simulink model "iter_imas_contr_4"  (Simulink 8.5)
settings: Solver=ode1  StartTime=EqTime  StopTime=1e8  FixedStep=SimStep  MaxStep=5.e-3  MinStep=2e-4  RelTol=1.e-3
undefined symbols (not defined in the file): Elong, g1, g1_term, g2, g2_term, g3, g3_term, g4, g4_term, g5, g5_term, g6, g6_term, Imax, key_imas, n_gaps, n_mc, ncam, npf, ntur, RupRd, scr_data, SimStep, Vcspf_up, vec_imas, volt
libraries: simulink x56
(part 2 of 3)

== system iter_imas_contr_4/kavin_contr/Control inputs 1/err(Ic) scr_data.dat/Icoil2 ref ==
  Time : Inport
  eob : Inport  Port=2
  Divide1 : Product  Inputs=**
  I1 : simulink/Lookup Tables/Lookup Table Dynamic  LookUpMeth=Interpolation-Use End Values  OutDataTypeStr=fixdt('double')  OutputDataTypeScalingMode=Specify via dialog  OutDataType=fixdt('double')  OutScaling=2^-10  DoSatur=off
  Memory2 : Memory
  c_eob : Switch  Threshold=1
  scr1 Read : DataStoreRead  DataStoreName=scr_data  DataStoreElements=scr_data(1,:)
  scr2 Read : DataStoreRead  DataStoreName=scr_data  DataStoreElements=scr_data(4,:)
  " " : Outport
  wires:
  c_eob/1 -> Memory2/1, Divide1/1
  Divide1/1 -> " "/1
  Time/1 -> I1/1
  eob/1 -> c_eob/2, Divide1/2
  Memory2/1 -> c_eob/3
  scr2 Read/1 -> I1/3
  I1/1 -> c_eob/1
  scr1 Read/1 -> I1/2

== system iter_imas_contr_4/kavin_contr/Control inputs 1/err(Ic) scr_data.dat/Icoil3 ref ==
  Time : Inport
  eob : Inport  Port=2
  Divide1 : Product  Inputs=**
  I1 : simulink/Lookup Tables/Lookup Table Dynamic  LookUpMeth=Interpolation-Use End Values  OutDataTypeStr=fixdt('double')  OutputDataTypeScalingMode=Specify via dialog  OutDataType=fixdt('double')  OutScaling=2^-10  DoSatur=off
  Memory2 : Memory
  c_eob : Switch  Threshold=1
  scr1 Read : DataStoreRead  DataStoreName=scr_data  DataStoreElements=scr_data(1,:)
  scr5 Read : DataStoreRead  DataStoreName=scr_data  DataStoreElements=scr_data(5,:)
  " " : Outport
  wires:
  c_eob/1 -> Memory2/1, Divide1/1
  Divide1/1 -> " "/1
  Time/1 -> I1/1
  eob/1 -> c_eob/2, Divide1/2
  Memory2/1 -> c_eob/3
  scr5 Read/1 -> I1/3
  I1/1 -> c_eob/1
  scr1 Read/1 -> I1/2

== system iter_imas_contr_4/kavin_contr/Control inputs 1/err(Ic) scr_data.dat/Icoil4 ref ==
  Time : Inport
  eob : Inport  Port=2
  Divide1 : Product  Inputs=**
  I1 : simulink/Lookup Tables/Lookup Table Dynamic  LookUpMeth=Interpolation-Use End Values  OutDataTypeStr=fixdt('double')  OutputDataTypeScalingMode=Specify via dialog  OutDataType=fixdt('double')  OutScaling=2^-10  DoSatur=off
  Memory2 : Memory
  c_eob : Switch  Threshold=1
  scr1 Read : DataStoreRead  DataStoreName=scr_data  DataStoreElements=scr_data(1,:)
  scr6 Read : DataStoreRead  DataStoreName=scr_data  DataStoreElements=scr_data(6,:)
  " " : Outport
  wires:
  c_eob/1 -> Memory2/1, Divide1/1
  Divide1/1 -> " "/1
  Time/1 -> I1/1
  eob/1 -> c_eob/2, Divide1/2
  Memory2/1 -> c_eob/3
  scr6 Read/1 -> I1/3
  I1/1 -> c_eob/1
  scr1 Read/1 -> I1/2

== system iter_imas_contr_4/kavin_contr/Control inputs 1/err(Ic) scr_data.dat/Icoil5 ref ==
  Time : Inport
  eob : Inport  Port=2
  Divide1 : Product  Inputs=**
  I1 : simulink/Lookup Tables/Lookup Table Dynamic  LookUpMeth=Interpolation-Use End Values  OutDataTypeStr=fixdt('double')  OutputDataTypeScalingMode=Specify via dialog  OutDataType=fixdt('double')  OutScaling=2^-10  DoSatur=off
  Memory2 : Memory
  c_eob : Switch  Threshold=1
  scr1 Read : DataStoreRead  DataStoreName=scr_data  DataStoreElements=scr_data(1,:)
  scr7 Read : DataStoreRead  DataStoreName=scr_data  DataStoreElements=scr_data(7,:)
  " " : Outport
  wires:
  c_eob/1 -> Memory2/1, Divide1/1
  Divide1/1 -> " "/1
  Time/1 -> I1/1
  eob/1 -> c_eob/2, Divide1/2
  Memory2/1 -> c_eob/3
  scr7 Read/1 -> I1/3
  I1/1 -> c_eob/1
  scr1 Read/1 -> I1/2

== system iter_imas_contr_4/kavin_contr/Control inputs 1/err(Ic) scr_data.dat/Icoil6 ref ==
  Time : Inport
  eob : Inport  Port=2
  Divide1 : Product  Inputs=**
  I1 : simulink/Lookup Tables/Lookup Table Dynamic  LookUpMeth=Interpolation-Use End Values  OutDataTypeStr=fixdt('double')  OutputDataTypeScalingMode=Specify via dialog  OutDataType=fixdt('double')  OutScaling=2^-10  DoSatur=off
  Memory2 : Memory
  c_eob : Switch  Threshold=1
  scr8 Read : DataStoreRead  DataStoreName=scr_data  DataStoreElements=scr_data(8,:)
  sct1 Read : DataStoreRead  DataStoreName=scr_data  DataStoreElements=scr_data(1,:)
  "  " : Outport
  wires:
  c_eob/1 -> Divide1/1, Memory2/1
  Divide1/1 -> "  "/1
  Time/1 -> I1/1
  eob/1 -> Divide1/2, c_eob/2
  Memory2/1 -> c_eob/3
  scr8 Read/1 -> I1/3
  I1/1 -> c_eob/1
  sct1 Read/1 -> I1/2

== system iter_imas_contr_4/kavin_contr/Control inputs 1/err(Ic) scr_data.dat/Icoil7 ref ==
  Time : Inport
  eob : Inport  Port=2
  Divide1 : Product  Inputs=**
  I1 : simulink/Lookup Tables/Lookup Table Dynamic  LookUpMeth=Interpolation-Use End Values  OutDataTypeStr=fixdt('double')  OutputDataTypeScalingMode=Specify via dialog  OutDataType=fixdt('double')  OutScaling=2^-10  DoSatur=off
  Memory2 : Memory
  c_eob : Switch  Threshold=1
  scr1 Read : DataStoreRead  DataStoreName=scr_data  DataStoreElements=scr_data(1,:)
  scr9 Read : DataStoreRead  DataStoreName=scr_data  DataStoreElements=scr_data(9,:)
  " " : Outport
  wires:
  c_eob/1 -> Divide1/1, Memory2/1
  Divide1/1 -> " "/1
  Time/1 -> I1/1
  eob/1 -> c_eob/2, Divide1/2
  Memory2/1 -> c_eob/3
  scr9 Read/1 -> I1/3
  I1/1 -> c_eob/1
  scr1 Read/1 -> I1/2

== system iter_imas_contr_4/kavin_contr/Control inputs 1/err(Ic) scr_data.dat/Icoil8 ref ==
  Time : Inport
  eob : Inport  Port=2
  Divide1 : Product  Inputs=**
  I1 : simulink/Lookup Tables/Lookup Table Dynamic  LookUpMeth=Interpolation-Use End Values  OutDataTypeStr=fixdt('double')  OutputDataTypeScalingMode=Specify via dialog  OutDataType=fixdt('double')  OutScaling=2^-10  DoSatur=off
  Memory2 : Memory
  c_eob : Switch  Threshold=1
  scr1 Read : DataStoreRead  DataStoreName=scr_data  DataStoreElements=scr_data(1,:)
  scr10 Read : DataStoreRead  DataStoreName=scr_data  DataStoreElements=scr_data(10,:)
  "  " : Outport
  wires:
  c_eob/1 -> Divide1/1, Memory2/1
  Divide1/1 -> "  "/1
  Time/1 -> I1/1
  eob/1 -> c_eob/2, Divide1/2
  Memory2/1 -> c_eob/3
  scr10 Read/1 -> I1/3
  I1/1 -> c_eob/1
  scr1 Read/1 -> I1/2

== system iter_imas_contr_4/kavin_contr/Control inputs 1/err(Ic) scr_data.dat/Icoil9 ref ==
  Time : Inport
  eob : Inport  Port=2
  Divide1 : Product  Inputs=**
  I1 : simulink/Lookup Tables/Lookup Table Dynamic  LookUpMeth=Interpolation-Use End Values  OutDataTypeStr=fixdt('double')  OutputDataTypeScalingMode=Specify via dialog  OutDataType=fixdt('double')  OutScaling=2^-10  DoSatur=off
  Memory2 : Memory
  c_eob : Switch  Threshold=1
  scr1 Read : DataStoreRead  DataStoreName=scr_data  DataStoreElements=scr_data(1,:)
  scr11 Read : DataStoreRead  DataStoreName=scr_data  DataStoreElements=scr_data(11,:)
  " " : Outport
  wires:
  c_eob/1 -> Divide1/1, Memory2/1
  Divide1/1 -> " "/1
  Time/1 -> I1/1
  eob/1 -> Divide1/2, c_eob/2
  Memory2/1 -> c_eob/3
  scr11 Read/1 -> I1/3
  I1/1 -> c_eob/1
  scr1 Read/1 -> I1/2

== system iter_imas_contr_4/kavin_contr/Control inputs 1/g1-g6.dat,g1_term-g6_term.dat/g1 ==
  Time : Inport
  eob : Inport  Port=2
  Memory1 : Memory
  Memory2 : Memory
  c_eob : Switch  Threshold=1
  "c_eob  " : Switch  Threshold=1
  c_eob  1 : Switch  Threshold=1
  g1 Read : DataStoreRead  DataStoreName=g1  DataStoreElements=g1(1,:)
  g1 Read1 : DataStoreRead  DataStoreName=g1  DataStoreElements=g1(2,:)
  g1_term,ref : Subsystem
  g1ref1 : simulink/Lookup Tables/Lookup Table Dynamic  LookUpMeth=Interpolation-Use End Values  OutDataTypeStr=fixdt('double')  OutputDataTypeScalingMode=Specify via dialog  OutDataType=fixdt('double')  OutScaling=2^-10  DoSatur=off
  Out1 : Outport
  wires:
  eob/1 -> "c_eob  "/2, c_eob/2, c_eob  1/2
  Memory1/1 -> "c_eob  "/3
  "c_eob  "/1 -> Memory1/1, g1_term,ref/3(Time_eob)
  g1_term,ref/1(Out1) -> c_eob/3
  c_eob/1 -> Out1/1
  Time/1 -> g1ref1/1, g1_term,ref/2(Time), "c_eob  "/1
  g1ref1/1 -> c_eob  1/1
  Memory2/1 -> c_eob  1/3
  c_eob  1/1 -> g1_term,ref/1(g1ref_eob), Memory2/1, c_eob/1
  g1 Read/1 -> g1ref1/2
  g1 Read1/1 -> g1ref1/3

== system iter_imas_contr_4/kavin_contr/Control inputs 1/g1-g6.dat,g1_term-g6_term.dat/g2 ==
  Time : Inport
  eob : Inport  Port=2
  Memory1 : Memory
  Memory2 : Memory
  c_eob : Switch  Threshold=1
  "c_eob  " : Switch  Threshold=1
  c_eob  1 : Switch  Threshold=1
  g2 Read : DataStoreRead  DataStoreName=g2  DataStoreElements=g2(1,:)
  g2 Read1 : DataStoreRead  DataStoreName=g2  DataStoreElements=g2(2,:)
  g2_term,ref : Subsystem
  g2ref : simulink/Lookup Tables/Lookup Table Dynamic  LookUpMeth=Interpolation-Use End Values  OutDataTypeStr=fixdt('double')  OutputDataTypeScalingMode=Specify via dialog  OutDataType=fixdt('double')  OutScaling=2^-10  DoSatur=off
  Out1 : Outport
  wires:
  eob/1 -> "c_eob  "/2, c_eob  1/2, c_eob/2
  Memory1/1 -> "c_eob  "/3
  "c_eob  "/1 -> g2_term,ref/3(Time_eob), Memory1/1
  g2_term,ref/1(Out1) -> c_eob/3
  c_eob/1 -> Out1/1
  g2 Read1/1 -> g2ref/3
  g2 Read/1 -> g2ref/2
  Time/1 -> g2ref/1, "c_eob  "/1, g2_term,ref/2(Time)
  g2ref/1 -> c_eob  1/1
  Memory2/1 -> c_eob  1/3
  c_eob  1/1 -> g2_term,ref/1(g2ref_eob), Memory2/1, c_eob/1

== system iter_imas_contr_4/kavin_contr/Control inputs 1/g1-g6.dat,g1_term-g6_term.dat/g3 ==
  Time : Inport
  eob : Inport  Port=2
  Memory1 : Memory
  Memory2 : Memory
  c_eob : Switch  Threshold=1
  "c_eob  " : Switch  Threshold=1
  c_eob  1 : Switch  Threshold=1
  g3 Read : DataStoreRead  DataStoreName=g3  DataStoreElements=g3(1,:)
  g3 Read1 : DataStoreRead  DataStoreName=g3  DataStoreElements=g3(2,:)
  g3_term,ref : Subsystem
  g3ref : simulink/Lookup Tables/Lookup Table Dynamic  LookUpMeth=Interpolation-Use End Values  OutDataTypeStr=fixdt('double')  OutputDataTypeScalingMode=Specify via dialog  OutDataType=fixdt('double')  OutScaling=2^-10  DoSatur=off
  Out1 : Outport
  wires:
  eob/1 -> "c_eob  "/2, c_eob/2, c_eob  1/2
  Memory1/1 -> "c_eob  "/3
  "c_eob  "/1 -> g3_term,ref/3(Time_eob), Memory1/1
  g3_term,ref/1(Out1) -> c_eob/3
  c_eob/1 -> Out1/1
  Time/1 -> g3ref/1, "c_eob  "/1, g3_term,ref/2(Time)
  g3ref/1 -> c_eob  1/1
  c_eob  1/1 -> g3_term,ref/1(g3ref_eob), Memory2/1, c_eob/1
  Memory2/1 -> c_eob  1/3
  g3 Read/1 -> g3ref/2
  g3 Read1/1 -> g3ref/3

== system iter_imas_contr_4/kavin_contr/Control inputs 1/g1-g6.dat,g1_term-g6_term.dat/g4 ==
  Time : Inport
  eob : Inport  Port=2
  Memory1 : Memory
  Memory2 : Memory
  c_eob : Switch  Threshold=1
  "c_eob  " : Switch  Threshold=1
  c_eob  1 : Switch  Threshold=1
  g4 Read : DataStoreRead  DataStoreName=g4  DataStoreElements=g4(1,:)
  g4 Read1 : DataStoreRead  DataStoreName=g4  DataStoreElements=g4(2,:)
  g4_term,ref : Subsystem
  g4ref : simulink/Lookup Tables/Lookup Table Dynamic  LookUpMeth=Interpolation-Use End Values  OutDataTypeStr=fixdt('double')  OutputDataTypeScalingMode=Specify via dialog  OutDataType=fixdt('double')  OutScaling=2^-10  DoSatur=off
  Out1 : Outport
  wires:
  eob/1 -> "c_eob  "/2, c_eob/2, c_eob  1/2
  Memory1/1 -> "c_eob  "/3
  "c_eob  "/1 -> Memory1/1, g4_term,ref/3(Time_eob)
  g4_term,ref/1(Out1) -> c_eob/3
  c_eob/1 -> Out1/1
  Time/1 -> g4ref/1, "c_eob  "/1, g4_term,ref/2(Time)
  g4ref/1 -> c_eob  1/1
  Memory2/1 -> c_eob  1/3
  c_eob  1/1 -> g4_term,ref/1(g4ref_eob), Memory2/1, c_eob/1
  g4 Read/1 -> g4ref/2
  g4 Read1/1 -> g4ref/3

== system iter_imas_contr_4/kavin_contr/Control inputs 1/g1-g6.dat,g1_term-g6_term.dat/g5 ==
  Time : Inport
  eob : Inport  Port=2
  Memory1 : Memory
  Memory2 : Memory
  c_eob : Switch  Threshold=1
  "c_eob  " : Switch  Threshold=1
  c_eob  1 : Switch  Threshold=1
  g5 Read : DataStoreRead  DataStoreName=g5  DataStoreElements=g5(1,:)
  g5 Read1 : DataStoreRead  DataStoreName=g5  DataStoreElements=g5(2,:)
  g5_term,ref : Subsystem
  g5ref : simulink/Lookup Tables/Lookup Table Dynamic  LookUpMeth=Interpolation-Use End Values  OutDataTypeStr=fixdt('double')  OutputDataTypeScalingMode=Specify via dialog  OutDataType=fixdt('double')  OutScaling=2^-10  DoSatur=off
  Out1 : Outport
  wires:
  eob/1 -> c_eob  1/2, "c_eob  "/2, c_eob/2
  Memory1/1 -> "c_eob  "/3
  "c_eob  "/1 -> Memory1/1, g5_term,ref/3(Time_eob)
  g5_term,ref/1(Out1) -> c_eob/3
  c_eob/1 -> Out1/1
  Time/1 -> g5ref/1, "c_eob  "/1, g5_term,ref/2(Time)
  g5ref/1 -> c_eob  1/1
  c_eob  1/1 -> Memory2/1, g5_term,ref/1(g5ref_eob), c_eob/1
  Memory2/1 -> c_eob  1/3
  g5 Read/1 -> g5ref/2
  g5 Read1/1 -> g5ref/3

== system iter_imas_contr_4/kavin_contr/Control inputs 1/g1-g6.dat,g1_term-g6_term.dat/g6 ==
  Time : Inport
  eob : Inport  Port=2
  Memory1 : Memory
  Memory2 : Memory
  c_eob : Switch  Threshold=1
  "c_eob  " : Switch  Threshold=1
  c_eob  1 : Switch  Threshold=1
  g6 Read : DataStoreRead  DataStoreName=g6  DataStoreElements=g6(1,:)
  g6 Read1 : DataStoreRead  DataStoreName=g6  DataStoreElements=g6(2,:)
  g6_term,ref : Subsystem
  g6ref : simulink/Lookup Tables/Lookup Table Dynamic  LookUpMeth=Interpolation-Use End Values  OutDataTypeStr=fixdt('double')  OutputDataTypeScalingMode=Specify via dialog  OutDataType=fixdt('double')  OutScaling=2^-10  DoSatur=off
  Out1 : Outport
  wires:
  eob/1 -> "c_eob  "/2, c_eob  1/2, c_eob/2
  Memory1/1 -> "c_eob  "/3
  "c_eob  "/1 -> Memory1/1, g6_term,ref/3(Time_eob)
  g6_term,ref/1(Out1) -> c_eob/3
  c_eob/1 -> Out1/1
  Time/1 -> g6ref/1, "c_eob  "/1, g6_term,ref/2(Time)
  g6ref/1 -> c_eob  1/1
  c_eob  1/1 -> g6_term,ref/1(g6ref_eob), Memory2/1, c_eob/1
  Memory2/1 -> c_eob  1/3
  g6 Read/1 -> g6ref/2
  g6 Read1/1 -> g6ref/3

== system iter_imas_contr_4/kavin_contr/Control inputs 1/trd/If Action Subsystem2 ==
  "time " : Inport
  Action Port : ActionPort  ActionType=then
  Data Store Write2 : DataStoreWrite  DataStoreName=trd
  wires:
  "time "/1 -> Data Store Write2/1

== system iter_imas_contr_4/kavin_contr/Control inputs 1/trd/Trigger ==
  Input : Inport
  Logical Operator : Logic  Operator=OR  AllPortsSameDT=off  OutDataTypeStr=float('double')
  Memory : Memory
  State : Outport
  wires:
  Memory/1 -> Logical Operator/2
  Input/1 -> Logical Operator/1
  Logical Operator/1 -> State/1, Memory/1

== system iter_imas_contr_4/kavin_contr/Control inputs 1/tterm/If Action Subsystem2 ==
  "time " : Inport
  Action Port : ActionPort  ActionType=then
  Data Store Write2 : DataStoreWrite  DataStoreName=tterm
  wires:
  "time "/1 -> Data Store Write2/1

== system iter_imas_contr_4/kavin_contr/Control inputs 1/tterm/Ip<cIp_end ==
  Ip : Inport
  Abs : Abs
  Data Store Read : DataStoreRead  DataStoreName=RupRd  DataStoreElements=RupRd(3)
  Relational Operator : RelationalOperator  Operator=<  OutDataTypeStr=boolean
  Out1 : Outport
  wires:
  Data Store Read/1 -> Abs/1
  Ip/1 -> Relational Operator/1
  Abs/1 -> Relational Operator/2
  Relational Operator/1 -> Out1/1

== system iter_imas_contr_4/kavin_contr/Control inputs 1/tterm/Trigger ==
  Input : Inport
  Logical Operator : Logic  Operator=OR  AllPortsSameDT=off  OutDataTypeStr=float('double')
  Memory : Memory
  State : Outport
  wires:
  Memory/1 -> Logical Operator/2
  Input/1 -> Logical Operator/1
  Logical Operator/1 -> State/1, Memory/1

== system iter_imas_contr_4/kavin_contr/Control1/VS control/Ip>cIp_end ==
  time : Inport
  Data Store Read2 : DataStoreRead  DataStoreName=tterm
  Relational Operator2 : RelationalOperator  Operator=<  OutDataTypeStr=float('double')
  1 or 0 : Outport
  wires:
  time/1 -> Relational Operator2/1
  Relational Operator2/1 -> 1 or 0/1
  Data Store Read2/1 -> Relational Operator2/2

== system iter_imas_contr_4/kavin_contr/Control1/VS control/dzdt noise1 ==
  VS3 inputs : Inport
  Time : Inport  Port=2
  Demux : Demux  Outputs=[1 1]
  Mux : Mux  Inputs=2
  Subsystem : Subsystem
  Sum2 : Sum
  Uniform Random Number : UniformRandomNumber  SampleTime=SimStep
  Out1 : Outport
  wires:
  VS3 inputs/1 -> Demux/1
  Demux/1 -> Sum2/2
  Sum2/1 -> Mux/1
  Demux/2 -> Mux/2
  Mux/1 -> Out1/1
  Uniform Random Number/1 -> Subsystem/1(Noise)
  Time/1 -> Subsystem/2(Time)
  Subsystem/1(Out1) -> Sum2/1

== system iter_imas_contr_4/kavin_contr/Control1/VS control/eob < 1 ==
  note: Ip<Ip_rd
  note: Ip>Ip_rd
  err VS : Inport
  Ip : Inport  Port=2
  "eob " : Inport  Port=3
  "time " : Inport  Port=4
  Compare To Constant1 : simulink/Logic and Bit Operations/Compare To Constant  relop=<  const=1  OutDataTypeStr=boolean  ZeroCross=off
  Divide1 : Product  Inputs=**
  Divide4 : Product  Inputs=**
  Ip < Ip_rd : Subsystem
  Ip > Ip_rd : Subsystem
  "Ip_rd " : Switch  Threshold=1
  Ip_rd tr : Subsystem
  VS. contr hl : Subsystem
  Out1 : Outport
  wires:
  Ip < Ip_rd/1(Out1) -> "Ip_rd "/1
  Ip > Ip_rd/1(Out1) -> "Ip_rd "/3
  Ip/1 -> Ip < Ip_rd/1(Ip), Ip > Ip_rd/1(Ip)
  Divide1/1 -> Out1/1
  VS. contr hl/1(Out1) -> Divide1/1
  "Ip_rd "/1 -> Divide1/2
  err VS/1 -> Divide4/1
  Divide4/1 -> VS. contr hl/1(In1)
  "eob "/1 -> Compare To Constant1/1, Ip_rd tr/2("eob ")
  Compare To Constant1/1 -> Divide4/2
  "time "/1 -> Ip_rd tr/1(Time)
  Ip_rd tr/1(0 or 1) -> "Ip_rd "/2

== system iter_imas_contr_4/kavin_contr/Control1/VS control/eob >= 1 ==
  Ipl : Inport
  time : Inport  Port=2
  err VS : Inport  Port=3
  Divide8 : Product  Inputs=**
  VS. contr1 : Subsystem
  dim or lim : Subsystem
  Out1 : Outport
  wires:
  err VS/1 -> VS. contr1/1(In1)
  Ipl/1 -> dim or lim/1(Ipl)
  time/1 -> dim or lim/2(Time)
  dim or lim/1(VS gain) -> Divide8/1
  VS. contr1/1(Out1) -> Divide8/2
  Divide8/1 -> Out1/1

== system iter_imas_contr_4/kavin_contr/Control1/VS control/t_tran2D ==
  Noise,VS3 : Inport
  Time : Inport  Port=2
  Data Store Read : DataStoreRead  DataStoreName=t_tran2D  DataStoreElements=t_tran2D
  Divide12 : Product  Inputs=**
  Relational Operator1 : RelationalOperator  Operator=>  OutDataTypeStr=float('double')
  Out1 : Outport
  wires:
  Noise,VS3/1 -> Divide12/1
  Time/1 -> Relational Operator1/1
  Data Store Read/1 -> Relational Operator1/2
  Relational Operator1/1 -> Divide12/2
  Divide12/1 -> Out1/1

== system iter_imas_contr_4/kavin_contr/Control1/controllers/ tt_kavin2.dat(1) ==
  Time : Inport
  1 : Constant
  Data Store Read : DataStoreRead  DataStoreName=ref_ramp  DataStoreElements=ref_ramp
  Data Store Read1 : DataStoreRead  DataStoreName=tdiv  DataStoreElements=tdiv
  Divide1 : Product  Inputs=/*
  Memory3 : Memory
  Relational Operator1 : RelationalOperator  OutDataTypeStr=float('double')
  Saturation1 : Saturate  UpperLimit=1  LowerLimit=0
  Subtract1 : Sum
  Subtract2 : Sum  Inputs=+-
  Subtract3 : Sum  Inputs=+-
  "switch1 " : Switch  Threshold=1
  1-0 : Outport
  0-1 : Outport  Port=2
  wires:
  "switch1 "/1 -> Memory3/1, Subtract2/1
  Memory3/1 -> "switch1 "/1
  Subtract2/1 -> Divide1/2
  Divide1/1 -> Subtract1/1
  Subtract1/1 -> Saturation1/1
  Saturation1/1 -> Subtract3/2, 1-0/1
  1/1 -> Subtract1/2, Subtract3/1
  Time/1 -> "switch1 "/3, Subtract2/2, Relational Operator1/1
  Data Store Read/1 -> Divide1/1
  Relational Operator1/1 -> "switch1 "/2
  Subtract3/1 -> 0-1/1
  Data Store Read1/1 -> Relational Operator1/2

== system iter_imas_contr_4/kavin_contr/Control1/controllers/Div rd contr ==
  gain : Inport
  time : Inport  Port=2
  err : Inport  Port=3
  Div_rd contr : Subsystem
  Divide3 : Product  Inputs=**
  Divide4 : Product  Inputs=**
  div_rd tr : Subsystem
  Div rd volt : Outport
  wires:
  gain/1 -> Divide3/1
  err/1 -> Divide4/2
  time/1 -> div_rd tr/1("time ")
  Divide3/1 -> Div rd volt/1
  Div_rd contr/1(Out1) -> Divide3/2
  Divide4/1 -> Div_rd contr/1(In1)
  div_rd tr/1(0 or 1) -> Divide4/1

== system iter_imas_contr_4/kavin_contr/Control1/controllers/Div. contr ==
  time : Inport
  err : Inport  Port=2
  gain : Inport  Port=3
  Div. contr. : Subsystem
  Divide : Product  Inputs=**
  Divide2 : Product  Inputs=**
  Udiv : Subsystem
  div tr : Subsystem
  "Div volt " : Outport
  wires:
  Udiv/1("Udiv ") -> "Div volt "/1
  Divide/1 -> Udiv/1(Udiv)
  div tr/1("0 or 1 ") -> Divide2/1
  Div. contr./1(Out1) -> Divide/1
  Divide2/1 -> Div. contr./1(In1)
  time/1 -> div tr/1(Time), Udiv/2("time ")
  err/1 -> Divide2/2
  gain/1 -> Divide/2

== system iter_imas_contr_4/kavin_contr/Control1/controllers/Ip>cIp_end1 ==
  Time : Inport
  1 : Constant
  "1 " : Switch  Threshold=1
  Data Store Read : DataStoreRead  DataStoreName=ref_ramp  DataStoreElements=ref_ramp
  Data Store Read2 : DataStoreRead  DataStoreName=tterm
  Divide4 : Product  Inputs=/*
  Memory1 : Memory
  Relational Operator2 : RelationalOperator  OutDataTypeStr=float('double')
  Saturation : Saturate  UpperLimit=1  LowerLimit=0
  Subtract1 : Sum  Inputs=-+
  Subtract2 : Sum  Inputs=+-
  Subtract3 : Sum
  1-0 : Outport
  0-1 : Outport  Port=2
  wires:
  Time/1 -> Subtract2/2, "1 "/3, Relational Operator2/1
  "1 "/1 -> Memory1/1, Subtract2/1
  Memory1/1 -> "1 "/1
  Subtract2/1 -> Divide4/2
  Divide4/1 -> Subtract3/1
  1/1 -> Subtract3/2, Subtract1/2
  Subtract3/1 -> Saturation/1
  Subtract1/1 -> 0-1/1
  Saturation/1 -> 1-0/1, Subtract1/1
  Data Store Read/1 -> Divide4/1
  Relational Operator2/1 -> "1 "/2
  Data Store Read2/1 -> Relational Operator2/2

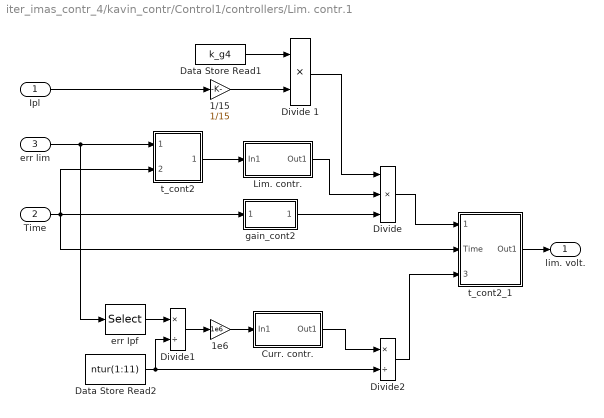
== system iter_imas_contr_4/kavin_contr/Control1/controllers/Lim. contr.1 ==
  Ipl : Inport
  Time : Inport  Port=2
  err lim : Inport  Port=3
  1/15 : Gain  Gain=1/15
  1e6 : Gain  Gain=1e6
  Curr. contr. : Subsystem
  Data Store Read1 : DataStoreRead  DataStoreName=k_g4  DataStoreElements=k_g4
  Data Store Read2 : DataStoreRead  DataStoreName=ntur  DataStoreElements=ntur(1:11)
  "Divide " : Product  Inputs=***
  Divide 1 : Product  Inputs=**
  Divide1 : Product  Inputs=*/
  Divide2 : Product  Inputs=*/
  Lim. contr. : Subsystem
  err Ipf : Selector  InputPortWidth=20  Indices=[9:19]
  gain_cont2 : Subsystem
  t_cont2 : Subsystem
  t_cont2_1 : Subsystem
  lim. volt. : Outport
  wires:
  err lim/1 -> err Ipf/1, t_cont2/1(errlim)
  Time/1 -> t_cont2_1/2(Time), gain_cont2/1(Time), t_cont2/2(Time)
  Divide1/1 -> 1e6/1
  Curr. contr./1(Out1) -> Divide2/1
  t_cont2/1(Out1) -> Lim. contr./1(In1)
  err Ipf/1 -> Divide1/1
  Data Store Read2/1 -> Divide1/2, Divide2/2
  "Divide "/1 -> t_cont2_1/1(lim. contr.)
  Divide2/1 -> t_cont2_1/3(Curr. cont.)
  t_cont2_1/1(Out1) -> lim. volt./1
  1e6/1 -> Curr. contr./1(In1)
  gain_cont2/1(Out1) -> "Divide "/3
  Lim. contr./1(Out1) -> "Divide "/2
  Ipl/1 -> 1/15/1
  Divide 1/1 -> "Divide "/1
  Data Store Read1/1 -> Divide 1/1
  1/15/1 -> Divide 1/2

== system iter_imas_contr_4/kavin_contr/Control1/controllers/curr term contr ==
  Time : Inport
  Icoil : Inport  Port=2
  " G_curr_term 1" : Gain  Gain=[zeros(8,11); eye(11); zeros(1,11)]  Multiplication=Matrix(K*u)
  Curr. term. contr : Subsystem
  Divide12 : Product  Inputs=**
  term tr : Subsystem
  term volt : Outport
  wires:
  Curr. term. contr/1(Out1) -> term volt/1
  Divide12/1 -> Curr. term. contr/1(In1)
  " G_curr_term 1"/1 -> Divide12/1
  Icoil/1 -> " G_curr_term 1"/1
  Time/1 -> term tr/1(Time)
  term tr/1(Out1) -> Divide12/2

== system iter_imas_contr_4/kavin_contr/Control1/controllers/div_divrd ==
  Time : Inport
  1 : Constant
  Data Store Read1 : DataStoreRead  DataStoreName=ref_ramp  DataStoreElements=ref_ramp
  Data Store Read2 : DataStoreRead  DataStoreName=trd
  Divide4 : Product  Inputs=/*
  Memory1 : Memory
  Relational Operator2 : RelationalOperator  OutDataTypeStr=float('double')
  Saturation : Saturate  UpperLimit=1  LowerLimit=0
  Subtract1 : Sum  Inputs=+-
  Subtract2 : Sum  Inputs=+-
  Subtract3 : Sum
  switch1 : Switch  Threshold=1
  1-0 : Outport
  0-1 : Outport  Port=2
  wires:
  switch1/1 -> Subtract2/1, Memory1/1
  Memory1/1 -> switch1/1
  Subtract2/1 -> Divide4/2
  Divide4/1 -> Subtract3/1
  Subtract3/1 -> Saturation/1
  Saturation/1 -> Subtract1/2, 1-0/1
  1/1 -> Subtract1/1, Subtract3/2
  Subtract1/1 -> 0-1/1
  Data Store Read1/1 -> Divide4/1
  Relational Operator2/1 -> switch1/2
  Time/1 -> Subtract2/2, switch1/3, Relational Operator2/1
  Data Store Read2/1 -> Relational Operator2/2

== system iter_imas_contr_4/kavin_contr/Control1/controllers/gain ==
  Ipl : Inport
  eob : Inport  Port=2
  " 1/15 " : Gain  Gain=1/15
  Data Store Read2 : DataStoreRead  DataStoreName=c_a_tpl2  DataStoreElements=c_a_tpl2
  Divide9 : Product  Inputs=**
  Saturation : Saturate  UpperLimit=1  LowerLimit=0
  c_eob : Switch  Threshold=1
  gain rd : Subsystem
  Out1 : Outport
  wires:
  Ipl/1 -> gain rd/2(Ipl), Divide9/2
  eob/1 -> c_eob/2, gain rd/1(eob)
  Data Store Read2/1 -> " 1/15 "/1
  " 1/15 "/1 -> Divide9/1
  Divide9/1 -> Saturation/1
  Saturation/1 -> c_eob/1
  gain rd/1(gain rd) -> c_eob/3
  c_eob/1 -> Out1/1

== system iter_imas_contr_4/kavin_contr/Control1/controllers/tt_kavin2.dat(1,4)1 ==
  Vdivrd : Inport
  Time : Inport  Port=2
  1 : Switch  Threshold=1
  Data Store Read : DataStoreRead  DataStoreName=tterm
  Memory1 : Memory
  Relational Operator : RelationalOperator  OutDataTypeStr=boolean
  "Vdivrd " : Outport
  wires:
  1/1 -> "Vdivrd "/1, Memory1/1
  Memory1/1 -> 1/1
  Vdivrd/1 -> 1/3
  Time/1 -> Relational Operator/1
  Data Store Read/1 -> Relational Operator/2
  Relational Operator/1 -> 1/2

== system iter_imas_contr_4/kavin_contr/Control1/volt.dat/tterm tr ==
  Time : Inport
  Data Store Read2 : DataStoreRead  DataStoreName=tterm
  Relational Operator2 : RelationalOperator  Operator=<  OutDataTypeStr=float('double')
  1 or 0 : Outport
  wires:
  Time/1 -> Relational Operator2/1
  Data Store Read2/1 -> Relational Operator2/2
  Relational Operator2/1 -> 1 or 0/1

== system iter_imas_contr_4/kavin_contr/Control1/volt.dat/volt1 ==
  Time : Inport
  0.001 : Gain  Gain=1e-3
  volt1 : simulink/Lookup Tables/Lookup Table Dynamic  LookUpMeth=Interpolation-Use End Values  OutDataTypeStr=fixdt('double')  OutputDataTypeScalingMode=Specify via dialog  OutDataType=fixdt('double')  OutScaling=2^-10  DoSatur=off
  volt1 Read : DataStoreRead  DataStoreName=volt  DataStoreElements=volt(1,:)
  volt2 Read : DataStoreRead  DataStoreName=volt  DataStoreElements=volt(2,:)
  Out1 : Outport
  wires:
  volt1 Read/1 -> 0.001/1
  volt1/1 -> Out1/1
  Time/1 -> volt1/1
  volt2 Read/1 -> volt1/3
  0.001/1 -> volt1/2

== system iter_imas_contr_4/kavin_contr/Control1/volt.dat/volt10 ==
  Time : Inport
  0.001 : Gain  Gain=1e-3
  volt1 : simulink/Lookup Tables/Lookup Table Dynamic  LookUpMeth=Interpolation-Use End Values  OutDataTypeStr=fixdt('double')  OutputDataTypeScalingMode=Specify via dialog  OutDataType=fixdt('double')  OutScaling=2^-10  DoSatur=off
  volt1 Read : DataStoreRead  DataStoreName=volt  DataStoreElements=volt(1,:)
  volt11 Read : DataStoreRead  DataStoreName=volt  DataStoreElements=volt(11,:)
  Out1 : Outport
  wires:
  volt1 Read/1 -> 0.001/1
  volt1/1 -> Out1/1
  Time/1 -> volt1/1
  volt11 Read/1 -> volt1/3
  0.001/1 -> volt1/2

== system iter_imas_contr_4/kavin_contr/Control1/volt.dat/volt11 ==
  Time : Inport
  0.001 : Gain  Gain=1e-3
  volt1 : simulink/Lookup Tables/Lookup Table Dynamic  LookUpMeth=Interpolation-Use End Values  OutDataTypeStr=fixdt('double')  OutputDataTypeScalingMode=Specify via dialog  OutDataType=fixdt('double')  OutScaling=2^-10  DoSatur=off
  volt1 Read : DataStoreRead  DataStoreName=volt  DataStoreElements=volt(1,:)
  volt12 Read : DataStoreRead  DataStoreName=volt  DataStoreElements=volt(12,:)
  Out1 : Outport
  wires:
  volt1 Read/1 -> 0.001/1
  volt1/1 -> Out1/1
  Time/1 -> volt1/1
  volt12 Read/1 -> volt1/3
  0.001/1 -> volt1/2

== system iter_imas_contr_4/kavin_contr/Control1/volt.dat/volt2 ==
  Time : Inport
  0.001 : Gain  Gain=1e-3
  volt1 : simulink/Lookup Tables/Lookup Table Dynamic  LookUpMeth=Interpolation-Use End Values  OutDataTypeStr=fixdt('double')  OutputDataTypeScalingMode=Specify via dialog  OutDataType=fixdt('double')  OutScaling=2^-10  DoSatur=off
  volt1 Read : DataStoreRead  DataStoreName=volt  DataStoreElements=volt(1,:)
  volt3 Read : DataStoreRead  DataStoreName=volt  DataStoreElements=volt(3,:)
  Out1 : Outport
  wires:
  volt1 Read/1 -> 0.001/1
  volt1/1 -> Out1/1
  Time/1 -> volt1/1
  volt3 Read/1 -> volt1/3
  0.001/1 -> volt1/2

== system iter_imas_contr_4/kavin_contr/Control1/volt.dat/volt3 ==
  Time : Inport
  0.001 : Gain  Gain=1e-3
  volt1 : simulink/Lookup Tables/Lookup Table Dynamic  LookUpMeth=Interpolation-Use End Values  OutDataTypeStr=fixdt('double')  OutputDataTypeScalingMode=Specify via dialog  OutDataType=fixdt('double')  OutScaling=2^-10  DoSatur=off
  volt1 Read : DataStoreRead  DataStoreName=volt  DataStoreElements=volt(1,:)
  volt4 Read : DataStoreRead  DataStoreName=volt  DataStoreElements=volt(4,:)
  Out1 : Outport
  wires:
  volt1 Read/1 -> 0.001/1
  volt1/1 -> Out1/1
  Time/1 -> volt1/1
  volt4 Read/1 -> volt1/3
  0.001/1 -> volt1/2

== system iter_imas_contr_4/kavin_contr/Control1/volt.dat/volt4 ==
  Time : Inport
  0.001 : Gain  Gain=1e-3
  volt1 : simulink/Lookup Tables/Lookup Table Dynamic  LookUpMeth=Interpolation-Use End Values  OutDataTypeStr=fixdt('double')  OutputDataTypeScalingMode=Specify via dialog  OutDataType=fixdt('double')  OutScaling=2^-10  DoSatur=off
  volt1 Read : DataStoreRead  DataStoreName=volt  DataStoreElements=volt(1,:)
  volt5 Read : DataStoreRead  DataStoreName=volt  DataStoreElements=volt(5,:)
  Out1 : Outport
  wires:
  volt1 Read/1 -> 0.001/1
  volt1/1 -> Out1/1
  Time/1 -> volt1/1
  volt5 Read/1 -> volt1/3
  0.001/1 -> volt1/2

== system iter_imas_contr_4/kavin_contr/Control1/volt.dat/volt5 ==
  Time : Inport
  0.001 : Gain  Gain=1e-3
  volt1 : simulink/Lookup Tables/Lookup Table Dynamic  LookUpMeth=Interpolation-Use End Values  OutDataTypeStr=fixdt('double')  OutputDataTypeScalingMode=Specify via dialog  OutDataType=fixdt('double')  OutScaling=2^-10  DoSatur=off
  volt1 Read : DataStoreRead  DataStoreName=volt  DataStoreElements=volt(1,:)
  volt6 Read : DataStoreRead  DataStoreName=volt  DataStoreElements=volt(6,:)
  Out1 : Outport
  wires:
  volt1 Read/1 -> 0.001/1
  volt1/1 -> Out1/1
  Time/1 -> volt1/1
  volt6 Read/1 -> volt1/3
  0.001/1 -> volt1/2

== system iter_imas_contr_4/kavin_contr/Control1/volt.dat/volt6 ==
  Time : Inport
  0.001 : Gain  Gain=1e-3
  volt1 : simulink/Lookup Tables/Lookup Table Dynamic  LookUpMeth=Interpolation-Use End Values  OutDataTypeStr=fixdt('double')  OutputDataTypeScalingMode=Specify via dialog  OutDataType=fixdt('double')  OutScaling=2^-10  DoSatur=off
  volt1 Read : DataStoreRead  DataStoreName=volt  DataStoreElements=volt(1,:)
  volt7 Read : DataStoreRead  DataStoreName=volt  DataStoreElements=volt(7,:)
  Out1 : Outport
  wires:
  volt1 Read/1 -> 0.001/1
  volt1/1 -> Out1/1
  Time/1 -> volt1/1
  volt7 Read/1 -> volt1/3
  0.001/1 -> volt1/2

== system iter_imas_contr_4/kavin_contr/Control1/volt.dat/volt7 ==
  Time : Inport
  0.001 : Gain  Gain=1e-3
  volt1 : simulink/Lookup Tables/Lookup Table Dynamic  LookUpMeth=Interpolation-Use End Values  OutDataTypeStr=fixdt('double')  OutputDataTypeScalingMode=Specify via dialog  OutDataType=fixdt('double')  OutScaling=2^-10  DoSatur=off
  volt1 Read : DataStoreRead  DataStoreName=volt  DataStoreElements=volt(1,:)
  volt8 Read : DataStoreRead  DataStoreName=volt  DataStoreElements=volt(8,:)
  Out1 : Outport
  wires:
  volt1 Read/1 -> 0.001/1
  volt1/1 -> Out1/1
  Time/1 -> volt1/1
  volt8 Read/1 -> volt1/3
  0.001/1 -> volt1/2

== system iter_imas_contr_4/kavin_contr/Control1/volt.dat/volt8 ==
  Time : Inport
  0.001 : Gain  Gain=1e-3
  volt1 : simulink/Lookup Tables/Lookup Table Dynamic  LookUpMeth=Interpolation-Use End Values  OutDataTypeStr=fixdt('double')  OutputDataTypeScalingMode=Specify via dialog  OutDataType=fixdt('double')  OutScaling=2^-10  DoSatur=off
  volt1 Read : DataStoreRead  DataStoreName=volt  DataStoreElements=volt(1,:)
  volt9 Read : DataStoreRead  DataStoreName=volt  DataStoreElements=volt(9,:)
  Out1 : Outport
  wires:
  volt1 Read/1 -> 0.001/1
  volt1/1 -> Out1/1
  Time/1 -> volt1/1
  volt9 Read/1 -> volt1/3
  0.001/1 -> volt1/2

== system iter_imas_contr_4/kavin_contr/Control1/volt.dat/volt9 ==
  Time : Inport
  0.001 : Gain  Gain=1e-3
  volt1 : simulink/Lookup Tables/Lookup Table Dynamic  LookUpMeth=Interpolation-Use End Values  OutDataTypeStr=fixdt('double')  OutputDataTypeScalingMode=Specify via dialog  OutDataType=fixdt('double')  OutScaling=2^-10  DoSatur=off
  volt1 Read : DataStoreRead  DataStoreName=volt  DataStoreElements=volt(1,:)
  volt10 Read : DataStoreRead  DataStoreName=volt  DataStoreElements=volt(10,:)
  Out1 : Outport
  wires:
  volt1 Read/1 -> 0.001/1
  volt1/1 -> Out1/1
  Time/1 -> volt1/1
  volt10 Read/1 -> volt1/3
  0.001/1 -> volt1/2

== system iter_imas_contr_4/kavin_contr/Control inputs 1/Err.1/tdiv if Ip is set /If Action  ==
  Time : Inport
  Action Port : ActionPort  ActionType=then
  Data Store Write19 : DataStoreWrite  DataStoreName=tdiv  DataStoreElements=tdiv
  wires:
  Time/1 -> Data Store Write19/1

== system iter_imas_contr_4/kavin_contr/Control inputs 1/g1-g6.dat,g1_term-g6_term.dat/g1/g1_term,ref ==
  g1ref_eob : Inport
  Time : Inport  Port=2
  Time_eob : Inport  Port=3
  Add2 : Sum
  Divide6 : Product  Inputs=**/
  Mux : Mux  Inputs=2
  RupRd Read : DataStoreRead  DataStoreName=RupRd  DataStoreElements=RupRd(2)
  Selector : Selector  NumberOfDimensions=2  InputPortWidth=13  IndexOptions=Index vector (dialog),Index vector (dialog)  Indices=2,2:50  OutputSizes=1,1
  Selector1 : Selector  NumberOfDimensions=2  InputPortWidth=13  IndexOptions=Index vector (dialog),Select all  Indices=1,1  OutputSizes=1,1
  g1_t Read : DataStoreRead  DataStoreName=g1_term  DataStoreElements=g1_term(:,:)
  g1_term,ref : simulink/Lookup Tables/Lookup Table Dynamic  LookUpMeth=Interpolation-Use End Values  OutDataTypeStr=fixdt('double')  OutputDataTypeScalingMode=Specify via dialog  OutDataType=fixdt('double')  OutScaling=2^-10  DoSatur=off
  trd Read : DataStoreRead  DataStoreName=trd_ref  DataStoreElements=trd_ref
  Out1 : Outport
  wires:
  g1_term,ref/1 -> Out1/1
  Time/1 -> g1_term,ref/1
  Add2/1 -> g1_term,ref/2
  Time_eob/1 -> Add2/1
  Selector/1 -> Mux/2
  Mux/1 -> g1_term,ref/3
  g1ref_eob/1 -> Mux/1
  Divide6/1 -> Add2/2
  Selector1/1 -> Divide6/1
  trd Read/1 -> Divide6/3
  RupRd Read/1 -> Divide6/2
  g1_t Read/1 -> Selector1/1, Selector/1

== system iter_imas_contr_4/kavin_contr/Control inputs 1/g1-g6.dat,g1_term-g6_term.dat/g2/g2_term,ref ==
  g2ref_eob : Inport
  Time : Inport  Port=2
  Time_eob : Inport  Port=3
  Add2 : Sum
  Divide6 : Product  Inputs=**/
  Mux : Mux  Inputs=2
  RupRd Read : DataStoreRead  DataStoreName=RupRd  DataStoreElements=RupRd(2)
  Selector : Selector  NumberOfDimensions=2  InputPortWidth=13  IndexOptions=Index vector (dialog),Index vector (dialog)  Indices=2,2:50  OutputSizes=1,1
  Selector1 : Selector  NumberOfDimensions=2  InputPortWidth=13  IndexOptions=Index vector (dialog),Select all  Indices=1,1  OutputSizes=1,1
  g2_t Read : DataStoreRead  DataStoreName=g2_term  DataStoreElements=g2_term(:,:)
  g2_term,ref : simulink/Lookup Tables/Lookup Table Dynamic  LookUpMeth=Interpolation-Use End Values  OutDataTypeStr=fixdt('double')  OutputDataTypeScalingMode=Specify via dialog  OutDataType=fixdt('double')  OutScaling=2^-10  DoSatur=off
  trd Read : DataStoreRead  DataStoreName=trd_ref  DataStoreElements=trd_ref
  Out1 : Outport
  wires:
  g2_term,ref/1 -> Out1/1
  Time/1 -> g2_term,ref/1
  Add2/1 -> g2_term,ref/2
  Time_eob/1 -> Add2/1
  Selector/1 -> Mux/2
  Mux/1 -> g2_term,ref/3
  g2ref_eob/1 -> Mux/1
  Divide6/1 -> Add2/2
  Selector1/1 -> Divide6/1
  trd Read/1 -> Divide6/3
  RupRd Read/1 -> Divide6/2
  g2_t Read/1 -> Selector/1, Selector1/1

== system iter_imas_contr_4/kavin_contr/Control inputs 1/g1-g6.dat,g1_term-g6_term.dat/g3/g3_term,ref ==
  g3ref_eob : Inport
  Time : Inport  Port=2
  Time_eob : Inport  Port=3
  Add2 : Sum
  Divide6 : Product  Inputs=**/
  Mux : Mux  Inputs=2
  RupRd Read : DataStoreRead  DataStoreName=RupRd  DataStoreElements=RupRd(2)
  Selector : Selector  NumberOfDimensions=2  InputPortWidth=13  IndexOptions=Index vector (dialog),Index vector (dialog)  Indices=2,2:50  OutputSizes=1,1
  Selector1 : Selector  NumberOfDimensions=2  InputPortWidth=13  IndexOptions=Index vector (dialog),Select all  Indices=1,1  OutputSizes=1,1
  g3_t Read : DataStoreRead  DataStoreName=g3_term  DataStoreElements=g3_term(:,:)
  g3_term,ref : simulink/Lookup Tables/Lookup Table Dynamic  LookUpMeth=Interpolation-Use End Values  OutDataTypeStr=fixdt('double')  OutputDataTypeScalingMode=Specify via dialog  OutDataType=fixdt('double')  OutScaling=2^-10  DoSatur=off
  trd Read : DataStoreRead  DataStoreName=trd_ref  DataStoreElements=trd_ref
  Out1 : Outport
  wires:
  g3_term,ref/1 -> Out1/1
  Time/1 -> g3_term,ref/1
  Add2/1 -> g3_term,ref/2
  Time_eob/1 -> Add2/1
  Selector/1 -> Mux/2
  Mux/1 -> g3_term,ref/3
  g3ref_eob/1 -> Mux/1
  Divide6/1 -> Add2/2
  Selector1/1 -> Divide6/1
  trd Read/1 -> Divide6/3
  RupRd Read/1 -> Divide6/2
  g3_t Read/1 -> Selector/1, Selector1/1

== system iter_imas_contr_4/kavin_contr/Control inputs 1/g1-g6.dat,g1_term-g6_term.dat/g4/g4_term,ref ==
  g4ref_eob : Inport
  Time : Inport  Port=2
  Time_eob : Inport  Port=3
  Add2 : Sum
  Divide6 : Product  Inputs=**/
  Mux : Mux  Inputs=2
  RupRd Read : DataStoreRead  DataStoreName=RupRd  DataStoreElements=RupRd(2)
  Selector : Selector  NumberOfDimensions=2  InputPortWidth=13  IndexOptions=Index vector (dialog),Index vector (dialog)  Indices=2,2:50  OutputSizes=1,1
  Selector1 : Selector  NumberOfDimensions=2  InputPortWidth=13  IndexOptions=Index vector (dialog),Select all  Indices=1,1  OutputSizes=1,1
  g4_t Read : DataStoreRead  DataStoreName=g4_term  DataStoreElements=g4_term(:,:)
  g4_term,ref : simulink/Lookup Tables/Lookup Table Dynamic  LookUpMeth=Interpolation-Use End Values  OutDataTypeStr=fixdt('double')  OutputDataTypeScalingMode=Specify via dialog  OutDataType=fixdt('double')  OutScaling=2^-10  DoSatur=off
  trd Read : DataStoreRead  DataStoreName=trd_ref  DataStoreElements=trd_ref
  Out1 : Outport
  wires:
  g4_term,ref/1 -> Out1/1
  Time/1 -> g4_term,ref/1
  Add2/1 -> g4_term,ref/2
  Time_eob/1 -> Add2/1
  Selector/1 -> Mux/2
  Mux/1 -> g4_term,ref/3
  g4ref_eob/1 -> Mux/1
  Divide6/1 -> Add2/2
  Selector1/1 -> Divide6/1
  trd Read/1 -> Divide6/3
  RupRd Read/1 -> Divide6/2
  g4_t Read/1 -> Selector/1, Selector1/1

== system iter_imas_contr_4/kavin_contr/Control inputs 1/g1-g6.dat,g1_term-g6_term.dat/g5/g5_term,ref ==
  g5ref_eob : Inport
  Time : Inport  Port=2
  Time_eob : Inport  Port=3
  Add2 : Sum
  Divide6 : Product  Inputs=**/
  Mux : Mux  Inputs=2
  RupRd Read : DataStoreRead  DataStoreName=RupRd  DataStoreElements=RupRd(2)
  Selector : Selector  NumberOfDimensions=2  InputPortWidth=13  IndexOptions=Index vector (dialog),Index vector (dialog)  Indices=2,2:50  OutputSizes=1,1
  Selector1 : Selector  NumberOfDimensions=2  InputPortWidth=13  IndexOptions=Index vector (dialog),Select all  Indices=1,1  OutputSizes=1,1
  g5_t Read : DataStoreRead  DataStoreName=g5_term  DataStoreElements=g5_term(:,:)
  g5_term,ref : simulink/Lookup Tables/Lookup Table Dynamic  LookUpMeth=Interpolation-Use End Values  OutDataTypeStr=fixdt('double')  OutputDataTypeScalingMode=Specify via dialog  OutDataType=fixdt('double')  OutScaling=2^-10  DoSatur=off
  trd Read : DataStoreRead  DataStoreName=trd_ref  DataStoreElements=trd_ref
  Out1 : Outport
  wires:
  g5_term,ref/1 -> Out1/1
  Time/1 -> g5_term,ref/1
  Add2/1 -> g5_term,ref/2
  Time_eob/1 -> Add2/1
  Mux/1 -> g5_term,ref/3
  g5ref_eob/1 -> Mux/1
  Divide6/1 -> Add2/2
  Selector1/1 -> Divide6/1
  trd Read/1 -> Divide6/3
  RupRd Read/1 -> Divide6/2
  Selector/1 -> Mux/2
  g5_t Read/1 -> Selector/1, Selector1/1

== system iter_imas_contr_4/kavin_contr/Control inputs 1/g1-g6.dat,g1_term-g6_term.dat/g6/g6_term,ref ==
  g6ref_eob : Inport
  Time : Inport  Port=2
  Time_eob : Inport  Port=3
  Add2 : Sum
  Divide6 : Product  Inputs=**/
  Mux : Mux  Inputs=2
  RupRd Read : DataStoreRead  DataStoreName=RupRd  DataStoreElements=RupRd(2)
  Selector : Selector  NumberOfDimensions=2  InputPortWidth=13  IndexOptions=Index vector (dialog),Index vector (dialog)  Indices=2,2:50  OutputSizes=1,1
  Selector1 : Selector  NumberOfDimensions=2  InputPortWidth=13  IndexOptions=Index vector (dialog),Select all  Indices=1,1  OutputSizes=1,1
  g6_t Read : DataStoreRead  DataStoreName=g6_term  DataStoreElements=g6_term(:,:)
  g6_term,ref : simulink/Lookup Tables/Lookup Table Dynamic  LookUpMeth=Interpolation-Use End Values  OutDataTypeStr=fixdt('double')  OutputDataTypeScalingMode=Specify via dialog  OutDataType=fixdt('double')  OutScaling=2^-10  DoSatur=off
  trd Read : DataStoreRead  DataStoreName=trd_ref  DataStoreElements=trd_ref
  Out1 : Outport
  wires:
  g6_term,ref/1 -> Out1/1
  Time/1 -> g6_term,ref/1
  Add2/1 -> g6_term,ref/2
  Time_eob/1 -> Add2/1
  Selector/1 -> Mux/2
  Mux/1 -> g6_term,ref/3
  g6ref_eob/1 -> Mux/1
  Divide6/1 -> Add2/2
  Selector1/1 -> Divide6/1
  trd Read/1 -> Divide6/3
  RupRd Read/1 -> Divide6/2
  g6_t Read/1 -> Selector/1, Selector1/1

== system iter_imas_contr_4/kavin_contr/Control1/VS control/dzdt noise1/Subsystem ==
  Noise : Inport
  Time : Inport  Port=2
  1.75 : Gain  Gain=1.75
  2e3 : Gain  Gain=2e3
  Data Store Read : DataStoreRead  DataStoreName=RupRd  DataStoreElements=RupRd(6)
  Difference : simulink/Discrete/Difference  ICPrevInput=0.0  InputProcessing=Inherited  OutMin=[]  OutMax=[]  OutDataType=sfix(16)  OutScaling=2^-10  DoSatur=off
  Divide1 : Product  Inputs=*/
  Divide11 : Product  Inputs=**
  Sqrt : Sqrt  SaturateOnIntegerOverflow=on
  Out1 : Outport
  wires:
  Time/1 -> Difference/1
  Noise/1 -> Divide11/1
  Data Store Read/1 -> 1.75/1
  1.75/1 -> Divide11/2
  2e3/1 -> Sqrt/1
  Difference/1 -> 2e3/1
  Divide1/1 -> Out1/1
  Divide11/1 -> Divide1/1
  Sqrt/1 -> Divide1/2

== system iter_imas_contr_4/kavin_contr/Control1/VS control/eob < 1/Ip < Ip_rd ==
  Ip : Inport
  " 1/15" : Gain  Gain=1/15
  1 : Constant
  Data Store Read : DataStoreRead  DataStoreName=c_a_tpl1_eob  DataStoreElements=c_a_tpl1_eob
  Data Store Read3 : DataStoreRead  DataStoreName=c_a_tpl_min  DataStoreElements=c_a_tpl_min
  Divide6 : Product  Inputs=**
  Saturation Dynamic : simulink/Discontinuities/Saturation Dynamic  OutMin=[]  OutMax=[]  OutDataTypeStr=Inherit: Same as second input  OutDataType=fixdt(1, 16)  OutScaling=2^-10  DoSatur=off
  Out1 : Outport
  wires:
  Data Store Read/1 -> " 1/15"/1
  " 1/15"/1 -> Divide6/1
  Data Store Read3/1 -> Saturation Dynamic/3
  Divide6/1 -> Saturation Dynamic/2
  Ip/1 -> Divide6/2
  Saturation Dynamic/1 -> Out1/1
  1/1 -> Saturation Dynamic/1

== system iter_imas_contr_4/kavin_contr/Control1/VS control/eob < 1/Ip > Ip_rd ==
  Ip : Inport
  1/15 : Gain  Gain=1/15
  3 : Constant
  Data Store Read2 : DataStoreRead  DataStoreName=c_a_tpl_min  DataStoreElements=c_a_tpl_min
  Saturation Dynamic1 : simulink/Discontinuities/Saturation Dynamic  OutMin=[]  OutMax=[]  OutDataTypeStr=Inherit: Same as second input  OutDataType=fixdt(1, 16)  OutScaling=2^-10  DoSatur=off
  Out1 : Outport
  wires:
  Saturation Dynamic1/1 -> Out1/1
  3/1 -> Saturation Dynamic1/1
  Data Store Read2/1 -> Saturation Dynamic1/3
  1/15/1 -> Saturation Dynamic1/2
  Ip/1 -> 1/15/1

== system iter_imas_contr_4/kavin_contr/Control1/VS control/eob < 1/Ip_rd tr ==
  Time : Inport
  "eob " : Inport  Port=2
  Compare To Constant1 : simulink/Logic and Bit Operations/Compare To Constant  relop=<  const=1  OutDataTypeStr=boolean  ZeroCross=off
  Compare To Constant2 : simulink/Logic and Bit Operations/Compare To Constant  relop=<  const=0  OutDataTypeStr=boolean  ZeroCross=off
  Data Store Read1 : DataStoreRead  DataStoreName=Ip_rd  DataStoreElements=Ip_rd
  Data Store Read2 : DataStoreRead  DataStoreName=trd
  Logical Operator1 : Logic  AllPortsSameDT=off  OutDataTypeStr=float('double')
  Logical Operator2 : Logic  Operator=OR  AllPortsSameDT=off  OutDataTypeStr=float('double')
  Relational Operator1 : RelationalOperator  OutDataTypeStr=float('double')
  0 or 1 : Outport
  wires:
  Data Store Read2/1 -> Relational Operator1/2
  Time/1 -> Relational Operator1/1
  Logical Operator2/1 -> 0 or 1/1
  Relational Operator1/1 -> Logical Operator2/1
  Data Store Read1/1 -> Compare To Constant2/1
  "eob "/1 -> Compare To Constant1/1
  Compare To Constant2/1 -> Logical Operator1/1
  Compare To Constant1/1 -> Logical Operator1/2
  Logical Operator1/1 -> Logical Operator2/2

== system iter_imas_contr_4/kavin_contr/Control1/VS control/eob < 1/VS. contr hl ==
  In1 : Inport
  " eye(20,2)" : Gain  Gain=eye(20,2)  Multiplication=Matrix(K*u)
  S-Function : S-Function  FunctionName=contr_vert_vs3  Parameters=2,2,2  SFunctionModules='contr_vert_vs3_wrapper'
  Selector : Selector  InputPortWidth=20  Indices=[2 1]
  Out1 : Outport
  wires:
  In1/1 -> " eye(20,2)"/1
  S-Function/1 -> Selector/1
  Selector/1 -> Out1/1
  " eye(20,2)"/1 -> S-Function/1

== system iter_imas_contr_4/kavin_contr/Control1/VS control/eob >= 1/VS. contr1 ==
  In1 : Inport
  " eye(20,2)" : Gain  Gain=eye(20,2)  Multiplication=Matrix(K*u)
  S-Function : S-Function  FunctionName=contr_vert_vs3  Parameters=2,2,1  SFunctionModules='contr_vert_vs3_wrapper'
  Selector : Selector  InputPortWidth=20  Indices=[2 1]
  Out1 : Outport
  wires:
  In1/1 -> " eye(20,2)"/1
  S-Function/1 -> Selector/1
  Selector/1 -> Out1/1
  " eye(20,2)"/1 -> S-Function/1

== system iter_imas_contr_4/kavin_contr/Control1/VS control/eob >= 1/dim or lim ==
  Ipl : Inport
  Time : Inport  Port=2
  1 : Constant  Value=0
  1/15 : Gain  Gain=1/15
  Data Store Read : DataStoreRead  DataStoreName=c_a_tpl1  DataStoreElements=c_a_tpl1
  Data Store Read1 : DataStoreRead  DataStoreName=tdiv  DataStoreElements=tdiv
  Data Store Read2 : DataStoreRead  DataStoreName=max_VS_lim  DataStoreElements=max_VS_lim
  Data Store Read3 : DataStoreRead  DataStoreName=RupRd  DataStoreElements=RupRd(4)
  Div : Product  Inputs=**
  Lim. Div. tr. : Switch  Threshold=1
  Relational Operator2 : RelationalOperator  OutDataTypeStr=float('double')
  Saturation Dynamic : simulink/Discontinuities/Saturation Dynamic  OutMin=[]  OutMax=[]  OutDataTypeStr=Inherit: Same as second input  OutDataType=fixdt(1, 16)  OutScaling=2^-10  DoSatur=off
  Saturation Dynamic1 : simulink/Discontinuities/Saturation Dynamic  OutMin=[]  OutMax=[]  OutDataTypeStr=Inherit: Same as second input  OutDataType=fixdt(1, 16)  OutScaling=2^-10  DoSatur=off
  VS gain : Outport
  wires:
  Lim. Div. tr./1 -> VS gain/1
  Saturation Dynamic/1 -> Lim. Div. tr./3
  Saturation Dynamic1/1 -> Lim. Div. tr./1
  Data Store Read/1 -> 1/15/1
  1/15/1 -> Div/2
  Div/1 -> Saturation Dynamic1/2, Saturation Dynamic/2
  Ipl/1 -> Div/1
  Relational Operator2/1 -> Lim. Div. tr./2
  1/1 -> Saturation Dynamic1/3, Saturation Dynamic/3
  Data Store Read2/1 -> Saturation Dynamic/1
  Time/1 -> Relational Operator2/1
  Data Store Read1/1 -> Relational Operator2/2
  Data Store Read3/1 -> Saturation Dynamic1/1

== system iter_imas_contr_4/kavin_contr/Control1/controllers/Div rd contr/Div_rd contr ==
  In1 : Inport
  S-Function : S-Function  FunctionName=contr_div  Parameters=20,n_mc,2  SFunctionModules='contr_curr_wrapper'
  Selector : Selector  InputPortWidth=20  Indices=[1:n_mc]
  Out1 : Outport
  wires:
  Selector/1 -> Out1/1
  In1/1 -> S-Function/1
  S-Function/1 -> Selector/1

== system iter_imas_contr_4/kavin_contr/Control1/controllers/Div rd contr/div_rd tr ==
  "time " : Inport
  Data Store Read2 : DataStoreRead  DataStoreName=trd
  Relational Operator2 : RelationalOperator  OutDataTypeStr=float('double')
  0 or 1 : Outport
  wires:
  Relational Operator2/1 -> 0 or 1/1
  "time "/1 -> Relational Operator2/1
  Data Store Read2/1 -> Relational Operator2/2

== system iter_imas_contr_4/kavin_contr/Control1/controllers/Div. contr/Div. contr. ==
  In1 : Inport
  S-Function : S-Function  FunctionName=contr_div  Parameters=20,n_mc,1  SFunctionModules='contr_div_wrapper'
  Selector : Selector  InputPortWidth=20  Indices=[1:n_mc]
  Out1 : Outport
  wires:
  Selector/1 -> Out1/1
  In1/1 -> S-Function/1
  S-Function/1 -> Selector/1

== system iter_imas_contr_4/kavin_contr/Control1/controllers/Div. contr/Udiv ==
  Udiv : Inport
  "time " : Inport  Port=2
  1 : Switch  Threshold=1
  Data Store Read2 : DataStoreRead  DataStoreName=trd
  Memory : Memory
  Relational Operator2 : RelationalOperator  OutDataTypeStr=float('double')
  "Udiv " : Outport
  wires:
  Udiv/1 -> 1/3
  Memory/1 -> 1/1
  1/1 -> Memory/1, "Udiv "/1
  Relational Operator2/1 -> 1/2
  "time "/1 -> Relational Operator2/1
  Data Store Read2/1 -> Relational Operator2/2

== system iter_imas_contr_4/kavin_contr/Control1/controllers/Div. contr/div tr ==
  Time : Inport
  Data Store Read2 : DataStoreRead  DataStoreName=tdiv  DataStoreElements=tdiv
  Relational Operator1 : RelationalOperator  OutDataTypeStr=float('double')
  "0 or 1 " : Outport
  wires:
  Relational Operator1/1 -> "0 or 1 "/1
  Time/1 -> Relational Operator1/1
  Data Store Read2/1 -> Relational Operator1/2

== system iter_imas_contr_4/kavin_contr/Control1/controllers/Lim. contr.1/Curr. contr. ==
  In1 : Inport
  Gain : Gain  Gain=eye(20,n_mc)  Multiplication=Matrix(K*u)
  S-Function : S-Function  FunctionName=contr_curr  Parameters=n_mc,n_mc,1  SFunctionModules='contr_curr_wrapper'
  Selector : Selector  InputPortWidth=20  Indices=[1:n_mc]
  Out1 : Outport
  wires:
  S-Function/1 -> Selector/1
  In1/1 -> Gain/1
  Selector/1 -> Out1/1
  Gain/1 -> S-Function/1

== system iter_imas_contr_4/kavin_contr/Control1/controllers/Lim. contr.1/Lim. contr. ==
  In1 : Inport
  S-Function : S-Function  FunctionName=contr_lim  Parameters=20,n_mc  SFunctionModules='contr_lim_wrapper'
  Selector : Selector  InputPortWidth=20  Indices=[1:n_mc]
  Out1 : Outport
  wires:
  In1/1 -> S-Function/1
  S-Function/1 -> Selector/1
  Selector/1 -> Out1/1
